simulink model "bms_csi"  (R2025a)
settings: Solver=FixedStepAuto  StartTime=0.0  StopTime=10.0  FixedStep=0.05  RelTol=1e-3
settings Model: ExtModeTrigDuration=100  Creator=adam  LastModifiedBy=adam

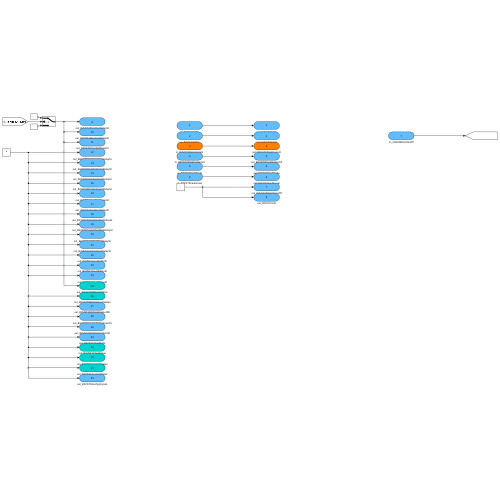
[thumbnail: Simulink's stored preview of the top-level diagram]
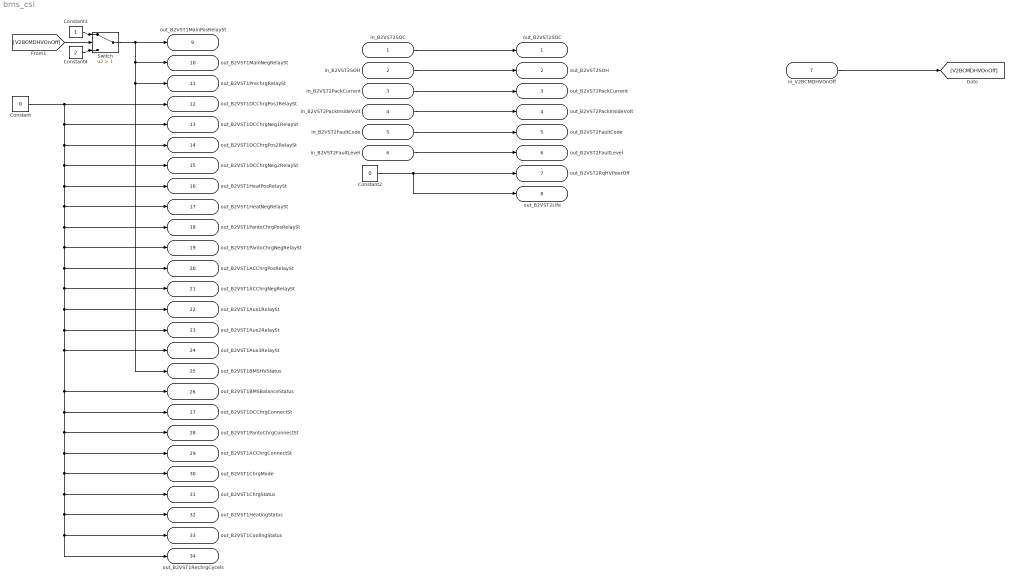
== system bms_csi ==
  in_B2VST2SOC : Inport
  in_B2VST2SOH : Inport  Port=2
  in_B2VST2PackCurrent : Inport  Port=3
  in_B2VST2PackInsideVolt : Inport  Port=4
  in_B2VST2FaultCode : Inport  Port=5
  in_B2VST2FaultLevel : Inport  Port=6
  in_V2BCMDHVOnOff : Inport  Port=7
  Constant : Constant  Value=0
  Constant2 : Constant  Value=0
  Constant3 : Constant
  Constant4 : Constant  Value=2
  Switch : Switch  Criteria=u2 > Threshold  Threshold=1  SaturateOnIntegerOverflow=off  InputSameDT=off
  out_B2VST2SOC : Outport
  out_B2VST2SOH : Outport  Port=2
  out_B2VST2PackCurrent : Outport  Port=3
  out_B2VST2PackInsideVolt : Outport  Port=4
  out_B2VST2FaultCode : Outport  Port=5
  out_B2VST2FaultLevel : Outport  Port=6
  out_B2VST2RqHVPoerOff : Outport  Port=7
  out_B2VST2Life : Outport  Port=8
  out_B2VST1MainPosRelaySt : Outport  Port=9
  out_B2VST1MainNegRelaySt : Outport  Port=10
  out_B2VST1PrechrgRelaySt : Outport  Port=11
  out_B2VST1DCChrgPos1RelaySt : Outport  Port=12
  out_B2VST1DCChrgNeg1RelaySt : Outport  Port=13
  out_B2VST1DCChrgPos2RelaySt : Outport  Port=14
  out_B2VST1DCChrgNeg2RelaySt : Outport  Port=15
  out_B2VST1HeatPosRelaySt : Outport  Port=16
  out_B2VST1HeatNegRelaySt : Outport  Port=17
  out_B2VST1PantoChrgPosRelaySt : Outport  Port=18
  out_B2VST1PantoChrgNegRelaySt : Outport  Port=19
  out_B2VST1ACChrgPosRelaySt : Outport  Port=20
  out_B2VST1ACChrgNegRelaySt : Outport  Port=21
  out_B2VST1Aux1RelaySt : Outport  Port=22
  out_B2VST1Aux2RelaySt : Outport  Port=23
  out_B2VST1Aux3RelaySt : Outport  Port=24
  out_B2VST1BMSHVStatus : Outport  Port=25
  out_B2VST1BMSBalanceStatus : Outport  Port=26
  out_B2VST1DCChrgConnectSt : Outport  Port=27
  out_B2VST1PantoChrgConnectSt : Outport  Port=28
  out_B2VST1ACChrgConnectSt : Outport  Port=29
  out_B2VST1ChrgMode : Outport  Port=30
  out_B2VST1ChrgStatus : Outport  Port=31
  out_B2VST1HeatingStatus : Outport  Port=32
  out_B2VST1CoolingStatus : Outport  Port=33
  out_B2VST1RechrgCycels : Outport  Port=34
  wires:
  in_B2VST2SOC/1 -> out_B2VST2SOC/1
  in_B2VST2FaultCode/1 -> out_B2VST2FaultCode/1
  Constant2/1 -> out_B2VST2Life/1, out_B2VST2RqHVPoerOff/1
  in_B2VST2PackInsideVolt/1 -> out_B2VST2PackInsideVolt/1
  in_B2VST2FaultLevel/1 -> out_B2VST2FaultLevel/1
  in_B2VST2SOH/1 -> out_B2VST2SOH/1
  in_B2VST2PackCurrent/1 -> out_B2VST2PackCurrent/1
  Constant/1 -> out_B2VST1ChrgStatus/1, out_B2VST1HeatingStatus/1, out_B2VST1CoolingStatus/1, out_B2VST1RechrgCycels/1, out_B2VST1ChrgMode/1, out_B2VST1ACChrgConnectSt/1, out_B2VST1PantoChrgConnectSt/1, out_B2VST1DCChrgConnectSt/1, out_B2VST1BMSBalanceStatus/1, out_B2VST1Aux3RelaySt/1, out_B2VST1Aux2RelaySt/1, out_B2VST1Aux1RelaySt/1, out_B2VST1ACChrgNegRelaySt/1, out_B2VST1ACChrgPosRelaySt/1, out_B2VST1PantoChrgNegRelaySt/1, out_B2VST1PantoChrgPosRelaySt/1, out_B2VST1HeatNegRelaySt/1, out_B2VST1HeatPosRelaySt/1, out_B2VST1DCChrgNeg2RelaySt/1, out_B2VST1DCChrgPos2RelaySt/1, out_B2VST1DCChrgNeg1RelaySt/1, out_B2VST1DCChrgPos1RelaySt/1
  in_V2BCMDHVOnOff/1 -> [V2BCMDHVOnOff]
  [V2BCMDHVOnOff] -> Switch/2
  Constant4/1 -> Switch/3
  Constant3/1 -> Switch/1
  Switch/1 -> out_B2VST1MainNegRelaySt/1, out_B2VST1PrechrgRelaySt/1, out_B2VST1BMSHVStatus/1, out_B2VST1MainPosRelaySt/1
